simulink model "transformfunc2"  (R2020b)
settings: Solver=VariableStepAuto  StartTime=0.0  StopTime=10.0  RelTol=1e-3
libraries: powerlib x17, powerlib_meascontrol x12
settings Model: Creator=admin  LastModifiedBy=admin

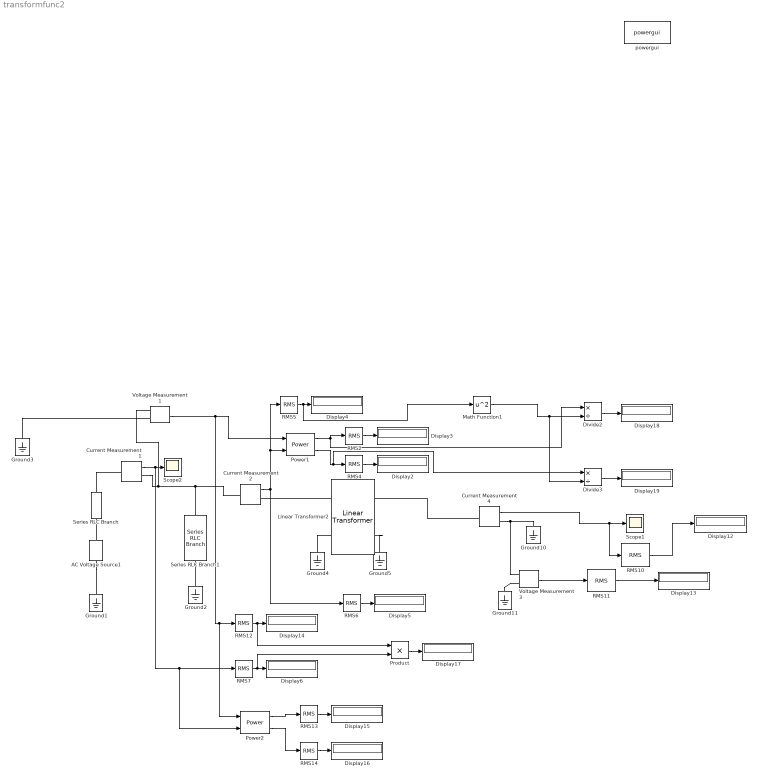
== system transformfunc2 ==
  AC Voltage Source1 : powerlib/Electrical Sources/AC Voltage Source  Amplitude=150*sqrt(2)  Phase=0  Frequency=50  SampleTime=0  Measurements=Voltage  BusType=swing  Pref=10e3  Qref=0  Qmin=-inf  Qmax=+inf
  Current Measurement1 : powerlib/Measurements/Current Measurement  PhasorSimulation=off  OutputType=Complex  PSBequivalent=0
  Current Measurement2 : powerlib/Measurements/Current Measurement  PhasorSimulation=off  OutputType=Complex  PSBequivalent=0
  Current Measurement4 : powerlib/Measurements/Current Measurement  PhasorSimulation=off  OutputType=Complex  PSBequivalent=0
  Display{2..6,12..19} (13 alike) : Display
  Divide2 : Product  Inputs=*/
  Divide3 : Product  Inputs=*/
  Ground{1..5,10..11} (7 alike) : powerlib/Elements/Ground  LConnTagsString=a
  Linear Transformer2 : powerlib/Elements/Linear Transformer  UNITS=SI  NominalPower=[250e6 50 ]  winding1=[2400 4.3218 0.45856]  winding2=[240 0.7938 0.084225]  ThreeWindings=off  winding3=[3.15e+05 0.7938 0.084225]  RmLm=[1.0805e+06 2866]  Measurements=None  DataType=on
  Math Function1 : Math  Operator=square  SaturateOnIntegerOverflow=on
  Power1 : powerlib_meascontrol/Measurements/Power  Freq=60  Vinit=[1, 0]  Iinit=[1, 0]  Ts=0
  Power2 : powerlib_meascontrol/Measurements/Power  Freq=60  Vinit=[1, 0]  Iinit=[1, 0]  Ts=0
  Product : Product
  RMS{2,4..7,10..14} (10 alike) : powerlib_meascontrol/Measurements/RMS  TrueRMS=on  Freq=50  RMSInit=0  Ts=0
  Scope1 : Scope
  Scope2 : Scope
  Series RLC Branch : powerlib/Elements/Series RLC Branch  LConnTagsString=__new0  RConnTagsString=__new0  BranchType=R  Resistance=100  Inductance=1e-3  SetiL0=off  InitialCurrent=0  Capacitance=1e-6  Setx0=off  InitialVoltage=0  Measurements=None
  Series RLC Branch1 : powerlib/Elements/Series RLC Branch  LConnTagsString=__new0  RConnTagsString=__new0  BranchType=RC  Resistance=1  Inductance=1e-3  SetiL0=off  InitialCurrent=0  Capacitance=1e-6  Setx0=off  InitialVoltage=0  Measurements=None
  Voltage Measurement1 : powerlib/Measurements/Voltage Measurement  PhasorSimulation=off  OutputType=Complex  PSBequivalent=0
  Voltage Measurement3 : powerlib/Measurements/Voltage Measurement  PhasorSimulation=off  OutputType=Complex  PSBequivalent=0
  powergui : powerlib/powergui  Priority=1  SimulationMode=Continuous  SampleTime=50e-6  frequency=60  Iterations=50  frequencyindice=50  Pbase=100e6  ErrMax=1e-4  UnitsV=kV  UnitsW=MW  buscounter=0  FunctionMessages=off  echomessages=off  EnableUseOfTLC=off  CurrentSourceSwitches=off  DisableSnubberDevices=off  DisableRonSwitches=off  DisableVfSwitches=off  DisplayEquations=off  AutomaticDiscreteSolvers=off  SolverType=Tustin/Backward Euler (TBE)  Interpol=off  ExternalGateDelay=off  methode=off  Ts=100  x0status=blocks  SPID=on  SwTol=0  HookPort=off  NonlinearTolerance=1e-4  nMaxIteration=100  ContinueOnMaxIteration=off  RestoreLinks=warning  ResistiveCurrentMeasurement=off  Frange=[0:2:500]  Ylog=off  Xlog=on  ShowGrid=off  save=off  variable=ZData  structure=0  ZoomFFT=off  StartTime=0.0  cycles=1  DisplayStyle=1  fundamental=60  FreqAxis=off  MaxFrequency=1000  frequencyindicesteady=1  RmsSteady=1  display=off
  wires:
  Current Measurement1/1 -> Power2/2, RMS7/1, Scope2/1
  RMS2/1 -> Display3/1
  Power1/2 -> Divide3/1, RMS4/1
  Power1/1 -> RMS2/1, Divide2/1
  Voltage Measurement1/1 -> Power2/1, RMS12/1, Power1/1
  RMS4/1 -> Display2/1
  RMS5/1 -> Math Function1/1, Display4/1
  Current Measurement2/1 -> RMS6/1, Power1/2, RMS5/1
  RMS6/1 -> Display5/1
  RMS7/1 -> Product/2, Display6/1
  RMS12/1 -> Product/1, Display14/1
  RMS13/1 -> Display15/1
  RMS14/1 -> Display16/1
  Power2/2 -> RMS14/1
  Power2/1 -> RMS13/1
  Product/1 -> Display17/1
  Divide2/1 -> Display18/1
  Math Function1/1 -> Divide3/2, Divide2/2
  Divide3/1 -> Display19/1
  Voltage Measurement3/1 -> RMS11/1
  RMS11/1 -> Display13/1
  RMS10/1 -> Display12/1
  Current Measurement4/1 -> RMS10/1, Scope1/1
  connections:
  AC Voltage Source1/LConn1 -- Ground1/LConn1
  AC Voltage Source1/RConn1 -- Series RLC Branch/RConn1
  Current Measurement1/LConn1 -- Series RLC Branch/LConn1
  Ground2/LConn1 -- Series RLC Branch1/RConn1
  Current Measurement1/RConn1 -- Series RLC Branch1/LConn1 -- Current Measurement2/LConn1 -- Voltage Measurement1/LConn1
  Voltage Measurement1/LConn2 -- Ground3/LConn1
  Linear Transformer2/LConn1 -- Current Measurement2/RConn1
  Linear Transformer2/LConn2 -- Ground4/LConn1
  Linear Transformer2/RConn2 -- Ground5/LConn1
  Current Measurement4/RConn1 -- Voltage Measurement3/LConn1 -- Ground10/LConn1
  Voltage Measurement3/LConn2 -- Ground11/LConn1
  Current Measurement4/LConn1 -- Linear Transformer2/RConn1
